simulink model "SatelliteADCS"  (R2019b)
settings: Solver=ode23tb  StartTime=0.0  StopTime=20  FixedStep=0.00005  RelTol=1e-3
undefined symbols (not defined in the file): IAU
libraries: sharedtransform x9, aerolibconvert2 x4, aerolibtransform2 x1, aerolibgravity2 x1, simulink_extras x1
settings Model: Creator=Dell  LastModifiedBy=as.safari
settings SolverCC: SolverResetMethod=Robust

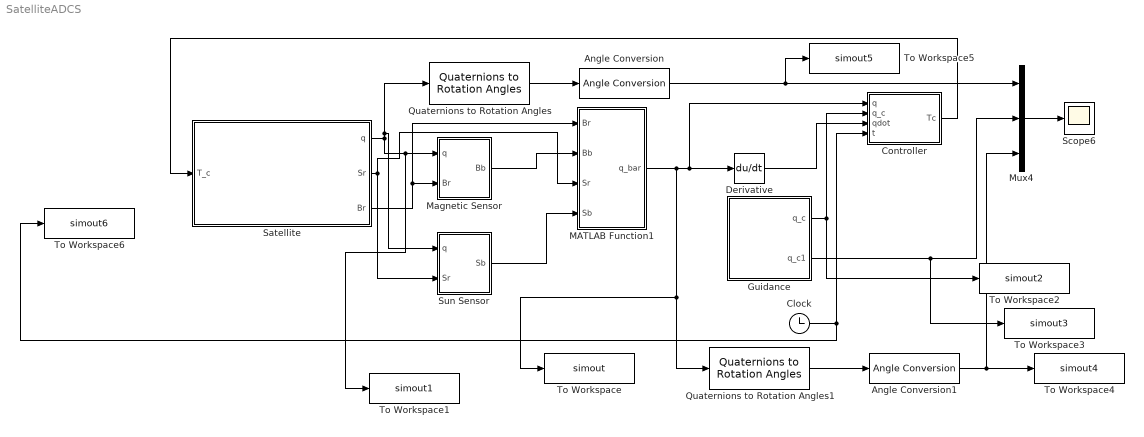
== system SatelliteADCS ==
  Angle Conversion : aerolibconvert2/Angle Conversion  IU=rad  OU=deg
  Angle Conversion1 : aerolibconvert2/Angle Conversion  IU=rad  OU=deg
  Clock : Clock
  Controller : MATLAB Function  TreatAsAtomicUnit=on
  Derivative : Derivative
  Guidance : Subsystem
  MATLAB Function1 : MATLAB Function  TreatAsAtomicUnit=on
  Magnetic Sensor : Subsystem
  Mux4 : Mux  Inputs=3
  Quaternions to Rotation Angles : sharedtransform/Quaternions to Rotation Angles  rotationOrder=ZYX  aMode=aMode
      settings: SourceProductBaseCode=AE
  Quaternions to Rotation Angles1 : sharedtransform/Quaternions to Rotation Angles  rotationOrder=ZYX  aMode=aMode
      settings: SourceProductBaseCode=AE
  "Satellite " : Subsystem  mask{J=[1000 0 0; 0 500 0; 0 0 700], phi0=0, psi0=deg2rad(0), theta0=0, p0=0, q0=0, r0=0}
      mask prompts: J "Inertia Matrix"
      mask init:
      | q0(1,1) = cos(psi0/2) * cos(theta0/2) * cos(phi0/2) ... 
      |     + sin(psi0/2) * sin(theta0/2) * sin(phi0/2);
      | q0(2,1) = cos(psi0/2) * cos(theta0/2) * sin(phi0/2) ... 
      |     - sin(psi0/2) * sin(theta0/2) * cos(phi0/2);
      | q0(3,1) = cos(psi0/2) * sin(theta0/2) * cos(phi0/2) ... 
      |     + sin(psi0/2) * cos(theta0/2) * sin(phi0/2);
      | q0(4,1) = sin(psi0/2) * cos(theta0/2) * cos(phi0/2) ... 
      |     - cos(psi0/2) * sin(theta0/2) * sin(phi0/2);
  Scope6 : Scope
  Sun Sensor : Subsystem
  To Workspace : ToWorkspace  VariableName=simout  SaveFormat=Timeseries  SampleTime=-1
  To Workspace1 : ToWorkspace  VariableName=simout1  SaveFormat=Timeseries  SampleTime=-1
  To Workspace2 : ToWorkspace  VariableName=simout2  SaveFormat=Timeseries  SampleTime=-1
  To Workspace3 : ToWorkspace  VariableName=simout3  SaveFormat=Timeseries  SampleTime=-1
  To Workspace4 : ToWorkspace  VariableName=simout4  SaveFormat=Timeseries  SampleTime=-1
  To Workspace5 : ToWorkspace  VariableName=simout5  SaveFormat=Timeseries  SampleTime=-1
  To Workspace6 : ToWorkspace  VariableName=simout6  SaveFormat=Timeseries  SampleTime=-1
  wires:
  Clock/1 -> Controller/4(t), To Workspace6/1
  Quaternions to Rotation Angles/1 -> Angle Conversion/1
  Guidance/2(q_c1) -> To Workspace3/1, Mux4/2
  Angle Conversion/1 -> To Workspace5/1, Mux4/1
  Guidance/1(q_c) -> Controller/2(q_c), To Workspace2/1
  Quaternions to Rotation Angles1/1 -> Angle Conversion1/1
  Derivative/1 -> Controller/3(qdot)
  Angle Conversion1/1 -> Mux4/3, To Workspace4/1
  Sun Sensor/1(Sb) -> MATLAB Function1/4(Sb)
  Controller/1(Tc) -> "Satellite "/1(T_c)
  Magnetic Sensor/1(Bb) -> MATLAB Function1/2(Bb)
  Mux4/1 -> Scope6/1
  "Satellite "/1(q) -> Quaternions to Rotation Angles/1, Sun Sensor/1(q), To Workspace1/1, Magnetic Sensor/1(q)
  MATLAB Function1/1(q_bar) -> Derivative/1, Controller/1(q), To Workspace/1, Quaternions to Rotation Angles1/1
  "Satellite "/2(Sr) -> MATLAB Function1/3(Sr), Sun Sensor/2(Sr)
  "Satellite "/3(Br) -> MATLAB Function1/1(Br), Magnetic Sensor/2(Br)

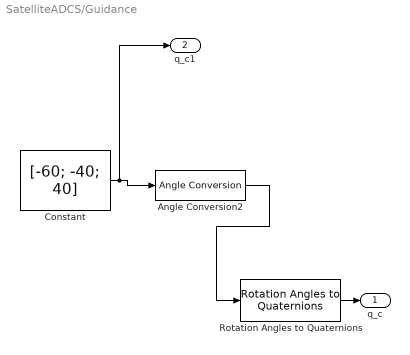
== system SatelliteADCS/Guidance ==
  Angle Conversion2 : aerolibconvert2/Angle Conversion  IU=deg  OU=rad
  Constant : Constant  Value=[-60; -40; 40]  VectorParams1D=off
  Rotation Angles to Quaternions : sharedtransform/Rotation Angles to Quaternions  rotationOrder=ZYX  aMode=aMode
      settings: SourceProductName=Aerospace Blockset  SourceProductBaseCode=AE
  q_c : Outport
  q_c1 : Outport  Port=2
  wires:
  Angle Conversion2/1 -> Rotation Angles to Quaternions/1
  Constant/1 -> q_c1/1, Angle Conversion2/1
  Rotation Angles to Quaternions/1 -> q_c/1

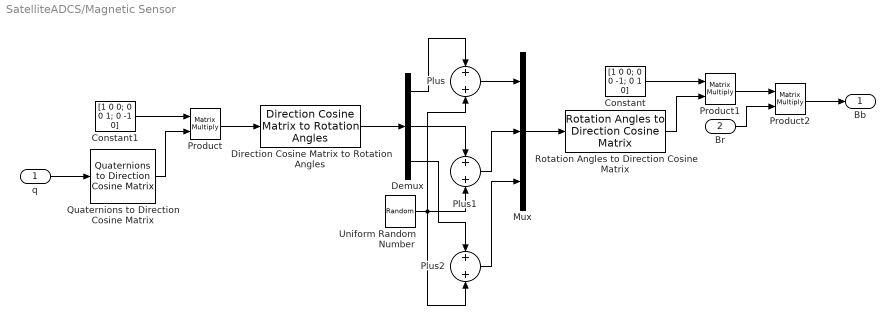
== system SatelliteADCS/Magnetic Sensor ==
  q : Inport
  Br : Inport  Port=2
  Constant : Constant  Value=[1 0 0; 0 0 -1; 0 1 0]
  Constant1 : Constant  Value=[1 0 0; 0 0 1; 0 -1 0]
  Demux : Demux  Outputs=3
  Direction Cosine Matrix to Rotation Angles : sharedtransform/Direction Cosine Matrix to Rotation Angles  rotationOrder=ZYX  aMode=aMode  action=None  tolerance=eps(2)
      settings: SourceProductName=Aerospace Blockset  SourceProductBaseCode=AE
  Mux : Mux  Inputs=3
  Plus : Sum
  Plus1 : Sum
  Plus2 : Sum
  Product : Product  Multiplication=Matrix(*)
  Product1 : Product  Multiplication=Matrix(*)
  Product2 : Product  Multiplication=Matrix(*)
  Quaternions to Direction Cosine Matrix : sharedtransform/Quaternions to  Direction Cosine Matrix  aMode=aMode
      settings: SourceProductName=Aerospace Blockset  SourceProductBaseCode=AE
  Rotation Angles to Direction Cosine Matrix : sharedtransform/Rotation Angles to Direction Cosine Matrix  rotationOrder=ZYX  aMode=aMode
      settings: SourceProductBaseCode=AE
  Uniform Random Number : UniformRandomNumber  Minimum=deg2rad(-0.5)  Maximum=deg2rad(0.5)  SampleTime=0.1
  Bb : Outport
  wires:
  Mux/1 -> Rotation Angles to Direction Cosine Matrix/1
  Product1/1 -> Product2/1
  Constant/1 -> Product1/1
  Quaternions to Direction Cosine Matrix/1 -> Product/2
  Product/1 -> Direction Cosine Matrix to Rotation Angles/1
  Demux/1 -> Plus/1
  Plus2/1 -> Mux/3
  Plus1/1 -> Mux/2
  Direction Cosine Matrix to Rotation Angles/1 -> Demux/1
  Rotation Angles to Direction Cosine Matrix/1 -> Product1/2
  Demux/2 -> Plus1/1
  Br/1 -> Product2/2
  Demux/3 -> Plus2/1
  Uniform Random Number/1 -> Plus/2, Plus1/2, Plus2/2
  Plus/1 -> Mux/1
  Constant1/1 -> Product/1
  q/1 -> Quaternions to Direction Cosine Matrix/1
  Product2/1 -> Bb/1

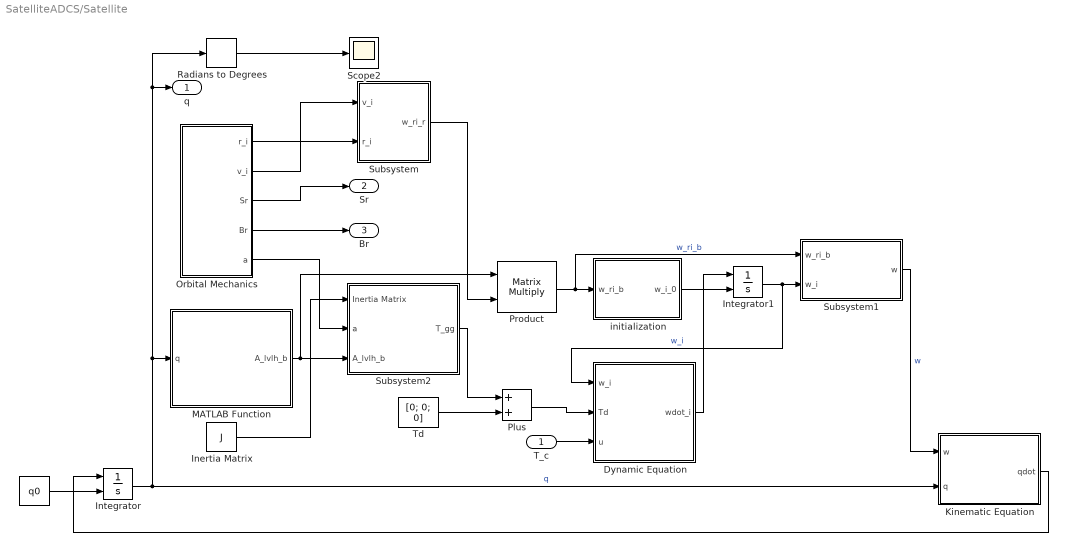
== system SatelliteADCS/Satellite  ==
  T_c : Inport
  " " : Constant  Value=q0  VectorParams1D=off
  Dynamic Equation : Subsystem
  "Inertia Matrix " : Constant  Value=J  VectorParams1D=off
  Integrator : Integrator  InitialConditionSource=external
  Integrator1 : Integrator  InitialConditionSource=external
  Kinematic Equation : Subsystem
  MATLAB Function : MATLAB Function  TreatAsAtomicUnit=on
  Orbital Mechanics : Subsystem  mask{r_a=800e3, r_p=800e3, i=deg2rad(75), w=deg2rad(0), Omega=deg2rad(0)}
      mask init:
      | G = 6.669 * 10^(-11);
      | M_Earth = 5.9742 * 10^24;
      | mu = G * M_Earth;
      | RE = 6378.15e3;
      | e = (r_a - r_p) / (r_a + r_p);
      | a = (r_a + r_p) / 2 +RE;
      | R0 = a;
      | n = sqrt(mu / R0^3);
  Plus : Sum
  Product : Product  Multiplication=Matrix(*)
  Radians to Degrees : simulink_extras/Transformations/Radians to Degrees
  Scope2 : Scope
  Subsystem : Subsystem
  Subsystem1 : Subsystem
  Subsystem2 : Subsystem
  Td : Constant  Value=[0; 0; 0]  VectorParams1D=off
  initialization : Subsystem
  q : Outport
  Sr : Outport  Port=2
  Br : Outport  Port=3  PortDimensions=[3,1]
  wires:
  "Inertia Matrix "/1 -> Subsystem2/1(Inertia Matrix)
  Orbital Mechanics/5(a) -> Subsystem2/2(a)
  " "/1 -> Integrator/2
  Kinematic Equation/1(qdot) -> Integrator/1
  Subsystem/1(w_ri_r) -> Product/2
  Orbital Mechanics/1(r_i) -> Subsystem/2("r_i ")
  Subsystem1/1(w) -> Kinematic Equation/1("w ")  "w"
  Dynamic Equation/1(wdot_i) -> Integrator1/1
  T_c/1 -> Dynamic Equation/3(u)
  initialization/1(w_i_0) -> Integrator1/2
  Subsystem2/1(T_gg) -> Plus/1
  Orbital Mechanics/3(Sr) -> Sr/1
  Td/1 -> Plus/2
  Radians to Degrees/1 -> Scope2/1
  Orbital Mechanics/2(v_i) -> Subsystem/1("v_i ")
  Product/1 -> initialization/1(w_ri_b), Subsystem1/1(w_ri_b)  "w_ri_b"
  Orbital Mechanics/4(Br) -> Br/1
  Plus/1 -> Dynamic Equation/2(Td)
  Integrator1/1 -> Subsystem1/2(w_i), Dynamic Equation/1("w_i ")  "w_i"
  Integrator/1 -> Radians to Degrees/1, q/1, MATLAB Function/1(q), Kinematic Equation/2(q)  "q"
  MATLAB Function/1(A_lvlh_b) -> Product/1, Subsystem2/3(A_lvlh_b)

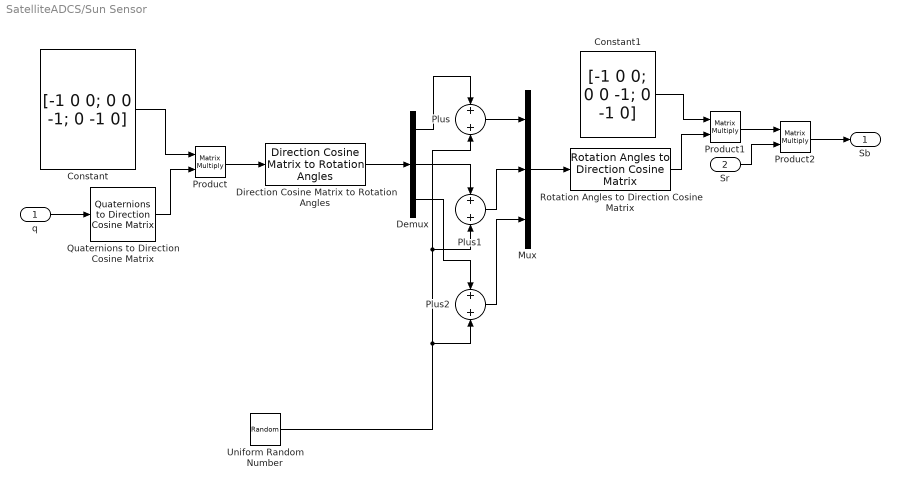
== system SatelliteADCS/Sun Sensor ==
  q : Inport
  Sr : Inport  Port=2
  Constant : Constant  Value=[-1 0 0; 0 0 -1; 0 -1 0]
  Constant1 : Constant  Value=[-1 0 0; 0 0 -1; 0 -1 0]
  Demux : Demux  Outputs=3
  Direction Cosine Matrix to Rotation Angles : sharedtransform/Direction Cosine Matrix to Rotation Angles  rotationOrder=ZYX  aMode=aMode  action=None  tolerance=eps(2)
      settings: SourceProductName=Aerospace Blockset  SourceProductBaseCode=AE
  Mux : Mux  Inputs=3
  Plus : Sum
  Plus1 : Sum
  Plus2 : Sum
  Product : Product  Multiplication=Matrix(*)
  Product1 : Product  Multiplication=Matrix(*)
  Product2 : Product  Multiplication=Matrix(*)
  Quaternions to Direction Cosine Matrix : sharedtransform/Quaternions to  Direction Cosine Matrix  aMode=aMode
      settings: SourceProductName=Aerospace Blockset  SourceProductBaseCode=AE
  Rotation Angles to Direction Cosine Matrix : sharedtransform/Rotation Angles to Direction Cosine Matrix  rotationOrder=ZYX  aMode=aMode
      settings: SourceProductBaseCode=AE
  Uniform Random Number : UniformRandomNumber  Minimum=deg2rad(-0.005)  Maximum=deg2rad(0.005)  SampleTime=0.1
  Sb : Outport
  wires:
  q/1 -> Quaternions to Direction Cosine Matrix/1
  Sr/1 -> Product2/2
  Product2/1 -> Sb/1
  Plus/1 -> Mux/1
  Rotation Angles to Direction Cosine Matrix/1 -> Product1/2
  Plus2/1 -> Mux/3
  Plus1/1 -> Mux/2
  Constant/1 -> Product/1
  Product1/1 -> Product2/1
  Quaternions to Direction Cosine Matrix/1 -> Product/2
  Constant1/1 -> Product1/1
  Demux/1 -> Plus/1
  Direction Cosine Matrix to Rotation Angles/1 -> Demux/1
  Mux/1 -> Rotation Angles to Direction Cosine Matrix/1
  Demux/2 -> Plus1/1
  Demux/3 -> Plus2/1
  Product/1 -> Direction Cosine Matrix to Rotation Angles/1
  Uniform Random Number/1 -> Plus/2, Plus1/2, Plus2/2

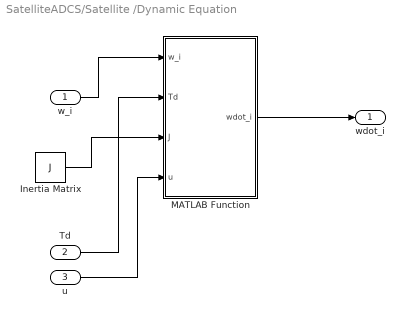
== system SatelliteADCS/Satellite /Dynamic Equation ==
  "w_i " : Inport
  Td : Inport  Port=2
  u : Inport  Port=3
  "Inertia Matrix " : Constant  Value=J  VectorParams1D=off
  MATLAB Function : MATLAB Function  TreatAsAtomicUnit=on
  wdot_i : Outport  PortDimensions=[3 1]
  wires:
  "w_i "/1 -> MATLAB Function/1(w_i)
  MATLAB Function/1(wdot_i) -> wdot_i/1
  u/1 -> MATLAB Function/4(u)
  Td/1 -> MATLAB Function/2(Td)
  "Inertia Matrix "/1 -> MATLAB Function/3(J)

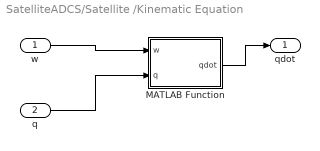
== system SatelliteADCS/Satellite /Kinematic Equation ==
  "w " : Inport  PortDimensions=[3 1]
  q : Inport  Port=2  PortDimensions=[4 1]
  MATLAB Function : MATLAB Function  TreatAsAtomicUnit=on
  qdot : Outport  PortDimensions=[4 1]
  wires:
  "w "/1 -> MATLAB Function/1(w)
  q/1 -> MATLAB Function/2(q)
  MATLAB Function/1(qdot) -> qdot/1

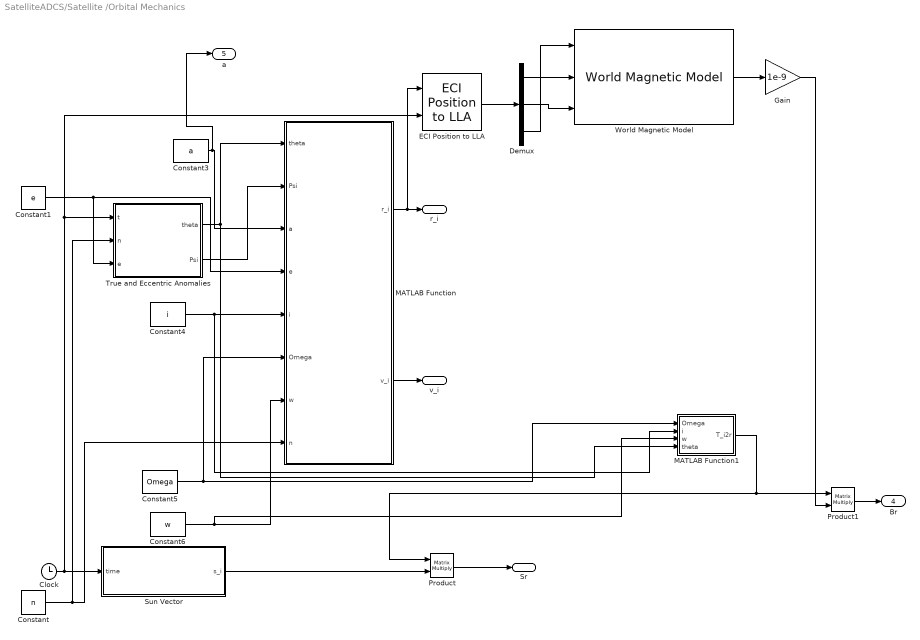
== system SatelliteADCS/Satellite /Orbital Mechanics ==
  Clock : Clock
  Constant : Constant  Value=n
  Constant1 : Constant  Value=e
  Constant3 : Constant  Value=a
  Constant4 : Constant  Value=i
  Constant5 : Constant  Value=Omega
  Constant6 : Constant  Value=w
  Demux : Demux  Outputs=3
  ECI Position to LLA : aerolibtransform2/ECI Position to LLA  red=IAU-2000/2006  year=2020  month=January  day=1  hour=0  min=0  sec=0  deltaT=Sec  errorflag=Error  extraparamflag=off  eunits=Metric (MKS)  earthmodel=WGS84  flat=1/298.257223563  eqradius=6378137
      settings: AttributesFormatString=%<red>  SourceProductName=Aerospace Blockset  SourceProductBaseCode=AE
  Gain : Gain  Gain=1e-9
  MATLAB Function : MATLAB Function  TreatAsAtomicUnit=on
  MATLAB Function1 : MATLAB Function  TreatAsAtomicUnit=on
  Product : Product  Multiplication=Matrix(*)
  Product1 : Product  Multiplication=Matrix(*)
  "Sun Vector " : Subsystem
  True and Eccentric Anomalies : MATLAB Function  TreatAsAtomicUnit=on
  World Magnetic Model : aerolibgravity2/World Magnetic Model  model=WMM2015 V2 (2015-2020)  customFile='WMM2015v2.COF'  units=Metric (MKS)  time_in=off  month=January  day=1  year=2020  action=Error  h_out=off  dec_out=off  inc_out=off  ti_out=off
      settings: SourceProductName=Aerospace Blockset  SourceProductBaseCode=AE
  r_i : Outport  PortDimensions=[3 1]
  v_i : Outport  Port=2  PortDimensions=[3 1]
  Sr : Outport  Port=3  PortDimensions=[3 1]
  Br : Outport  Port=4
  a : Outport  Port=5
  wires:
  Product1/1 -> Br/1
  MATLAB Function/1(r_i) -> r_i/1, ECI Position to LLA/1
  MATLAB Function/2(v_i) -> v_i/1
  World Magnetic Model/1 -> Gain/1
  Constant3/1 -> a/1, MATLAB Function/3(a)
  Demux/3 -> World Magnetic Model/1
  Demux/2 -> World Magnetic Model/3
  Demux/1 -> World Magnetic Model/2
  ECI Position to LLA/1 -> Demux/1
  Product/1 -> Sr/1
  Constant1/1 -> True and Eccentric Anomalies/3(e), MATLAB Function/4(e)
  True and Eccentric Anomalies/2(Psi) -> MATLAB Function/2(Psi)
  Gain/1 -> Product1/2
  Constant/1 -> True and Eccentric Anomalies/2(n), MATLAB Function/8(n)
  Clock/1 -> True and Eccentric Anomalies/1(t), ECI Position to LLA/2, "Sun Vector "/1("time ")
  True and Eccentric Anomalies/1(theta) -> MATLAB Function1/4(theta), MATLAB Function/1(theta)
  Constant6/1 -> MATLAB Function1/3(w), MATLAB Function/7(w)
  Constant5/1 -> MATLAB Function1/1(Omega), MATLAB Function/6(Omega)
  Constant4/1 -> MATLAB Function1/2(i), MATLAB Function/5(i)
  "Sun Vector "/1(s_i) -> Product/2
  MATLAB Function1/1(T_i2r) -> Product/1, Product1/1

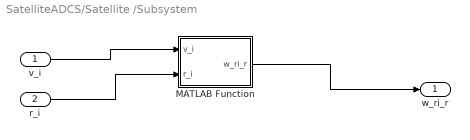
== system SatelliteADCS/Satellite /Subsystem ==
  "v_i " : Inport
  "r_i " : Inport  Port=2
  MATLAB Function : MATLAB Function  TreatAsAtomicUnit=on
  w_ri_r : Outport  PortDimensions=[3 1]
  wires:
  MATLAB Function/1(w_ri_r) -> w_ri_r/1
  "v_i "/1 -> MATLAB Function/1(v_i)
  "r_i "/1 -> MATLAB Function/2(r_i)

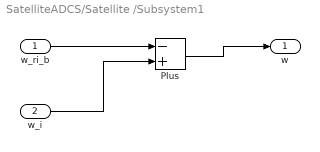
== system SatelliteADCS/Satellite /Subsystem1 ==
  w_ri_b : Inport  PortDimensions=[3 1]
  w_i : Inport  Port=2
  Plus : Sum  Inputs=-+
  w : Outport
  wires:
  w_ri_b/1 -> Plus/1
  w_i/1 -> Plus/2
  Plus/1 -> w/1

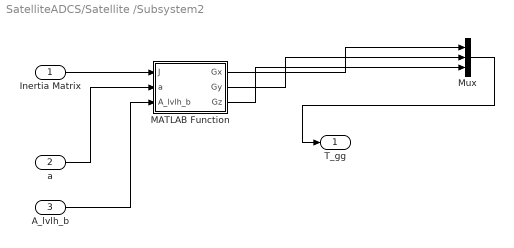
== system SatelliteADCS/Satellite /Subsystem2 ==
  Inertia Matrix : Inport
  a : Inport  Port=2
  A_lvlh_b : Inport  Port=3
  MATLAB Function : MATLAB Function  TreatAsAtomicUnit=on
  Mux : Mux  Inputs=3
  T_gg : Outport  PortDimensions=[3,1]
  wires:
  a/1 -> MATLAB Function/2(a)
  A_lvlh_b/1 -> MATLAB Function/3(A_lvlh_b)
  Inertia Matrix/1 -> MATLAB Function/1(J)
  MATLAB Function/2(Gy) -> Mux/2
  MATLAB Function/1(Gx) -> Mux/1
  MATLAB Function/3(Gz) -> Mux/3
  Mux/1 -> T_gg/1

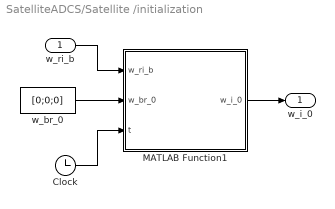
== system SatelliteADCS/Satellite /initialization ==
  w_ri_b : Inport
  Clock : Clock
  MATLAB Function1 : MATLAB Function  TreatAsAtomicUnit=on
  "w_br_0 " : Constant  Value=[0;0;0]  VectorParams1D=off
  w_i_0 : Outport  PortDimensions=[3 1]
  wires:
  "w_br_0 "/1 -> MATLAB Function1/2(w_br_0)
  w_ri_b/1 -> MATLAB Function1/1(w_ri_b)
  Clock/1 -> MATLAB Function1/3(t)
  MATLAB Function1/1(w_i_0) -> w_i_0/1

== system SatelliteADCS/Satellite /Orbital Mechanics/Sun Vector  ==
  "time " : Inport
  Julian Date Conversion : aerolibconvert2/Julian Date Conversion  year=2020  month=January  day=1  hour=00  min=00  sec=0  modflag=off  deltaT=Sec  errorflag=Error
      settings: SourceProductName=Aerospace Blockset  SourceProductBaseCode=AE
  "Sun Vector Model " : MATLAB Function  TreatAsAtomicUnit=on
  s_i : Outport  PortDimensions=[3 1]
  wires:
  Julian Date Conversion/1 -> "Sun Vector Model "/1(u)
  "Sun Vector Model "/1(y) -> s_i/1
  "time "/1 -> Julian Date Conversion/1

== matlab function SatelliteADCS/Satellite /Orbital Mechanics/MATLAB Function ==
  data: theta input; r_i output; v_i output; Psi input; a input; e input; i input; Omega input; w input; n input
function [r_i, v_i] = fcn(theta, Psi, a, e, i, Omega, w, n)
x = a * cos(Psi) - a * e;
y = a * sin(Psi) * sqrt(1 - e^2);
r = norm([x; y; 0]);
v_x = (a^2 * n)/r * (-sin(Psi));
v_y = (a^2 * n)/r * (sqrt(1 - e^2) * cos(Psi));
T_p2i = [cos(Omega) sin(Omega) 0; -sin(Omega) cos(Omega) 0; 0 0 1]' * [1 0 0; 0 cos(i) sin(i); 0 -sin(i) cos(i)]' * [cos(w) sin(w) 0; -sin(w) cos(w) 0; 0 0 1]';
[r_i] = T_p2i * [x; y; 0];
[v_i] = T_p2i * [v_x; v_y; 0];

== matlab function SatelliteADCS/Satellite /Orbital Mechanics/True and Eccentric Anomalies ==
  data: t input; n input; e input; theta output; Psi output
function [theta, Psi]  = fcn(t, n, e)

t_0 = 0;

%Mean Anomaly (t_0 = 0)
M = n*(t-t_0);

%Eccentric Anomaly (can use this method since e<1)
Psi_old= 0;
Psi_new = M;

while abs(Psi_new-Psi_old)>1e-12    
    Psi_old = Psi_new;
    Psi_new = M + e * sin(Psi_old);
end

Psi=Psi_new;

%True Anomaly
theta = 2*atan2(sqrt(1+e)*tan(Psi/2),sqrt(1-e));

if theta<0
    theta = theta+2*pi;
end

== matlab function SatelliteADCS/Satellite /Subsystem2/MATLAB Function ==
  data: J input; Gx output; a input; A_lvlh_b input; Gy output; Gz output
function [Gx, Gy, Gz]  = fcn(J, a, A_lvlh_b)
G = 6.669 * 10^(-11);
M_Earth = 5.9742 * 10^24;
mu = G * M_Earth;
% G = 6*mu/(2*a^3) * [q1 * (Iz - Iy); q2 * (Iz - Ix); 0];
% Gx = 3*mu/(2*R0^3) * (Iz - Iy) * sin(2*phi) * cos(theta)^2;
% Gy = 3*mu/(2*R0^3) * (Iz - Ix) * sin(2*theta) * cos(phi);
% Gz = 3*mu/(2*R0^3) * (Ix - Iy) * sin(2*theta) * sin(phi);
R = A_lvlh_b * [0;0;-a];
x = 3 * mu / a^5 * R;
y = J * R;
G = cross(x,y);
Gx = G(1);
Gy = G(2);
Gz = G(3);

== matlab function SatelliteADCS/Satellite /Orbital Mechanics/Sun Vector /Sun Vector Model  ==
  data: u input; y output
function y = fcn(u)
JD_TU1 = u;
T_UT1 = (JD_TU1 - 2451545.0)/36525;
Lambda_Mo = 280.460 + 36000.771 * T_UT1;
Lambda_Mo = rem(Lambda_Mo, 360);
if Lambda_Mo < 0
    Lambda_Mo =  Lambda_Mo + 360; 
end
T_TDB = T_UT1;
Mo = 357.5291092 + 35999.05034 * T_TDB;
Mo = rem(Mo, 360);
if Mo < 0
    Mo = Mo + 360;
end
Lambda_ecliptic = Lambda_Mo + 1.914666471 * sind(Mo) + 0.019994643 * sind(2 * Mo);
ro = 1.000140612 - 0.016708617 * cosd(Mo) - 0.000139589 * cosd(2 * Mo);
epsilon = 23.439291 - 0.0130042 * T_TDB;
AU = 149597870 * 1000   ;
r_bar_o = [ro * cosd(Lambda_ecliptic) , ro * cosd(epsilon) * sind(Lambda_ecliptic), ro * sind(epsilon) * sind(Lambda_ecliptic)] * AU;
y = r_bar_o';

== matlab function SatelliteADCS/Satellite /Subsystem/MATLAB Function ==
  data: v_i input; w_ri_r output; r_i input
function w_ri_r = fcn(v_i,  r_i)
    % Keplerian Orbit
    w_i = 0;
    r = norm(r_i);
    w_j = -1/(r^2 * norm(cross(v_i,r_i))) * dot(v_i, dot(r_i,v_i)*r_i - r^2*v_i);
    w_k = 0;
    w_ri_r = [w_i ; w_j; w_k];

== matlab function SatelliteADCS/Satellite /MATLAB Function ==
  data: q input; A_lvlh_b output
function A_lvlh_b = fcn(q)
q0 = q(1);
q1 = q(2);
q2 = q(3);
q3 = q(4);
A_lvlh_b = [2*q0^2 - 1 + 2*q1^2, 2*q1*q2 + 2*q0*q3, 2*q1*q3 - 2*q0*q2; ...
    2*q1*q2 - 2*q0*q3, 2*q0^2 - 1 + 2*q2^2, 2*q2*q3 + 2*q0*q1; ...
    2*q1*q3 + 2*q0*q2, 2*q2*q3 - 2*q0*q1, 2*q0^2 - 1 + 2*q3^2];

== matlab function SatelliteADCS/Satellite /Kinematic Equation/MATLAB Function ==
  data: w input; qdot output; q input
function qdot = fcn(w, q)
% w1 = w(1);
% w2 = w(2);
% w3 = w(3);
% qdot = 1/2 * [ 0 -w1 -w2 -w3; ...    
%               w1  0   w3 -w2; ...
%               w2 -w3  0   w1; ...
%               w3  w2 -w1  0 ] * q;
q0 = q(1);
q1 = q(2);
q2 = q(3);
q3 = q(4);
qdot = 1/2 * [q0 -q1 -q2 -q3; q1 q0 -q3 q2; q2 q3 q0 -q1; q3 -q2 q1 q0] * [0;w];

== matlab function SatelliteADCS/Satellite /Dynamic Equation/MATLAB Function ==
  data: w_i input; Td input; J input; wdot_i output; u input
function wdot_i = fcn(w_i, Td, J, u)
wdot_i = inv(J) * (cross(-w_i, (J * w_i)) + Td + u);

== matlab function SatelliteADCS/Satellite /initialization/MATLAB Function1 ==
  data: w_ri_b input; w_br_0 input; t input; w_i_0 output
function w_i_0  = fcn(w_ri_b, w_br_0, t)
    if t == 0
        w_i_0 = w_br_0 + w_ri_b;
    else 
        w_i_0 = [0; 0; 0];
    end

== matlab function SatelliteADCS/Satellite /Orbital Mechanics/MATLAB Function1 ==
  data: Omega input; T_i2r output; i input; w input; theta input
function T_i2r = fcn(Omega, i, w, theta)
T_i2p = [cos(w) sin(w) 0; -sin(w) cos(w) 0; 0 0 1] ...
    * [1 0 0; 0 cos(i) sin(i); 0 -sin(i) cos(i)] ...
    * [cos(Omega) sin(Omega) 0; -sin(Omega) cos(Omega) 0; 0 0 1];
T_p2r = [-sin(theta) cos(theta) 0; 0 0 -1; -cos(theta) sin(theta) 0];
T_i2r = T_i2p * T_p2r;

== matlab function SatelliteADCS/Controller ==
  data: q input; q_c input; Tc output; qdot input; t input
function Tc = fcn(q, q_c, qdot, t)
if t <= 1
    Tc = [0;0;0];
else
    qT4 = q_c(1);
    qT1 = q_c(2);
    qT2 = q_c(3);
    qT3 = q_c(4);
    qS4 = q(1);
    qS2 = q(3);
    qS3 = q(4);
    qS1 = q(2);
    qdot4 = qdot(1);
    qdot1 = qdot(2);
    qdot2 = qdot(3);
    qdot3 = qdot(4);
    w = 2 * [qS4 qS3 -qS2 -qS1; -qS3 qS4 qS1 -qS2; qS2 -qS1 qS4 -qS3] * ...
        [qdot1; qdot2; qdot3; qdot4];
    q_E = [qT4 qT3 -qT2 qT1; -qT3 qT4 qT1 qT2; qT2 -qT1 qT4 qT3; -qT1 -qT2 -qT3 qT4] ...
        * [-qS1; -qS2; -qS3; qS4];
    p = w(1);
    q = w(2);
    r = w(3);
    Kx = 1000;
    Ky = 2000;
    Kz = 500;
    Kxd = -1000;
    Kyd = -700;
    Kzd = -1400;
    Tcx = 2 * Kx * q_E(1) * q_E(4) + Kxd * p;
    Tcy = 2 * Ky * q_E(2) * q_E(4) + Kyd * q;
    Tcz = 2 * Kz * q_E(3) * q_E(4) + Kzd * r;
    Tc = [Tcx; Tcy; Tcz];
end

== matlab function SatelliteADCS/MATLAB Function1 ==
  data: Br input; q_bar output; Bb input; Sr input; Sb input
function q_bar  = fcn(Br, Bb, Sr, Sb)
Br = Br / norm(Br);
Bb = Bb / norm(Bb);
Sr = Sr / norm(Sr);
Sb = Sb / norm(Sb);
wk = [1 10];
B = wk(1) * Br * Bb' + wk(2) * Sr * Sb';
S = B + B';
Z = [B(3,2) - B(2,3); B(1,3) - B(3,1); B(2,1) - B(1,2)];
sigma = trace(B);
K = [S - sigma*eye(3,3) Z; Z' sigma];
[V,D] = eig(K);
DE = real([D(1,1); D(2,2); D(3,3); D(4,4)]);
sig_max = max(DE);
if sig_max == DE(1)
    q_bar = [real(V(4,1));real(V(1:3,1))];
elseif sig_max == DE(2)
    q_bar = [real(V(4,2));real(V(1:3,2))];
elseif sig_max == DE(3)
    q_bar = [real(V(4,3));real(V(1:3,3))];
else
    q_bar = [real(V(4,4));real(V(1:3,4))];
end
